simulink model "CubeX_LQR_2D"  (R2016b)
settings: Solver=FixedStepDiscrete  StartTime=0.0  StopTime=inf  FixedStep=0.002  RelTol=1e-3
PreLoadFcn:
  | waijung.modelPreload; % Required for working with Waijung Blockset. Do not remove.
InitFcn:
  | cubeparameters
values from neighbouring files (symbols this model uses):
  A = [0 0 0 0 0 0 0 0 0 0 283.190307038 0 ... (36 elements, 6x6)]    [K_lqr_3D.mat]
  C = [1 0 0 0 0 0 0 1 0 0 0 0 ... (36 elements, 6x6)]    [K_lqr_3D.mat]
  deg_ = 0.0174532925199    [K_lqr_3D.mat]
  g = 9.81    [K_lqr_3D.mat]
  imu =     [K_lqr_3D.mat]
  K_lqr = [204.402503892 25.7626324054]    [K_lqr_3D.mat]
  motor =     [K_lqr_3D.mat]
undefined symbols (not defined in the file or in its folder): Link, LQFP100, ST, STM32F407VG, STM32F4DISCOVERY
libraries: simulink x39, stm32f4_i2c_lib x8, stm32f4_io_lib x7, cube_lib x5, BC_USB x2, stm32f4_adc_lib x1, stm32f4_device_config_lib x1
(part 1 of 3)
CloseFcn:
  | waijung.modelClose; % Required for working with Waijung Blockset. Do not remove.
settings Model: Creator=Hi  LastModifiedBy=Wall
settings DataIOCC: LimitDataPoints=on  SaveFormat=Array
settings OptimizationCC: LifeSpan=1
settings DebuggingCC: AllowSymbolicDim=off  SFUnexpectedBacktrackingDiag=warning  SFNoUnconditionalDefaultTransitionDiag=warning  SFExecutionAtInitializationDiag=none
settings HardwareCC: ProdBitPerPointer=32  ProdBitPerSizeT=32  ProdBitPerPtrDiffT=32  ProdLargestAtomicFloat=None  ProdIntDivRoundTo=Undefined  ProdWordSize=32  ProdHWDeviceType=ARM Compatible->Cortex - M4  TargetEndianess=LittleEndian  TargetHWDeviceType=ARM Compatible->Cortex - M4
settings ModelReferenceCC: PropagateSignalLabelsOutOfModel=off
settings RTWCC: SystemTargetFile=stm32f4.tlc  GenerateMakefile=off  TemplateMakefile=ert_default_tmf  Description=STM32F4 Target
settings CodeAppCC: ForceParamTrailComments=on  IgnoreCustomStorageClasses=off  OperatorAnnotations=on  SimulinkDataObjDesc=on  InsertBlockDesc=on  MATLABSourceComments=on
settings STFCustomTargetCC: ModelReferenceCompliant=off  CombineOutputUpdateFcns=on  ERTCustomFileBanners=on  SupportContinuousTime=off  SupportNonInlinedSFcns=off  RemoveResetFunc=on  MATLABClassNameForMDSCustomization=Simulink.SoftwareTarget.ERTCustomization  GRTInterface=off  SystemTargetFile=stm32f4.tlc
settings ERTTargetCC: ModelReferenceCompliant=off  ParMdlRefBuildCompliant=off  CompOptLevelCompliant=off  ConcurrentExecutionCompliant=off  ERTFirstTimeCompliant=off  ModelStepFunctionPrototypeControlCompliant=off  CPPClassGenCompliant=off  UseToolchainInfoCompliant=off  ERTSrcFileBannerTemplate=stm32f4_code_template.cgt  ERTHdrFileBannerTemplate=stm32f4_code_template.cgt  ERTDataSrcFileTemplate=stm32f4_code_template.cgt  ERTDataHdrFileTemplate=stm32f4_code_template.cgt  ERTCustomFileTemplate=stm32f4_file_process.tlc  ConvertIfToSwitch=off  SuppressUnreachableDefaultCases=off
settings ConfigComp: CovMetricSettings=dw  CovHtmlReporting=on  CovSaveCumulativeToWorkspaceVar=on  CovSaveSingleToWorkspaceVar=on  CovExternalEMLEnable=off

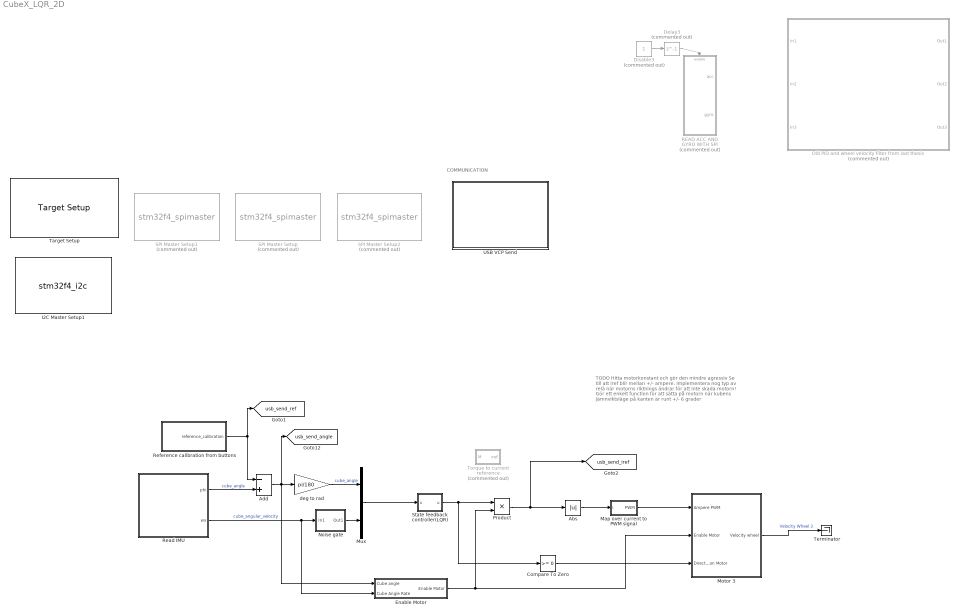
== system CubeX_LQR_2D ==
  note: TODO
      | Hitta motorkonstant och gör den mindre agressiv
      | Se till att iref blir mellan +/- ampere.
      |
      | Implementera nog typ av relä när motorns riktnings
      | ändrar för att inte skada motorn!
      |
      | Gör ett enkelt function för att sätta på motorn när kubens
      | jämnviktsläge på kanten är runt +/- 6 grader
  note: COMMUNICATION
  Abs : Abs
  Add : Sum  Inputs=-+
  Compare To Zero : simulink/Logic and Bit Operations/Compare To Zero  relop=>=  OutDataTypeStr=boolean
  Delay3 : Delay  Commented=on  DelayLength=1  InitialCondition=0
  Disable3 : Constant  Commented=on
  Enable Motor : Subsystem
  I2C Master Setup1 : S-Function  FunctionName=stm32f4_i2c  Parameters=configuration,module,transfer,clkspeed,timeout,sdapin,sclpin,writecount,readcount,inputtypearray,outputtypearray,confstr,sampletime,sampletimestr,blockid  SFunctionDeploymentMode=off  EnableBusSupport=off  mask(stm32f4_i2c){configuration=Setup, module=1, lastmodule=1, transfer=Blocking, dutycycle=TLow/THigh = 2, clkspeed=400, timeout=25, writecount=0, readcount=0, sdapin=B9, sclpin=B6, waitwritetime=0, inputtypearray=[0], outputtypearray=[0], confstr=["B","9","B","6","1","1","6","0","I2C_DutyCycle_2","0","off"], sampletime=-1, sampletimestr=0.002, blockid=I2CMasterSetup1}
      mask prompts: module "I2C Module"; lastmodule "Last module"; transfer "Transfer mode"; dutycycle "Duty cycle in fast mode"; clkspeed "Clock speed (kHz)"; timeout "Timeout (ms)"; writecount "Bytes write count"; readcount "Bytes read count"; sdapin "SDA pin"; sclpin "SCL pin"; waitwritetime "Wait write time (ms), default is 0"; inputtypearray "Input type array"; outputtypearray "Output type array"; confstr "Configuration string"; sampletime "Sample time (sec)"; sampletimestr "Compiled sample time (sec) in string"
      mask init:
      | stm32f4_i2c_callback('init');
      mask Help: web(fullfile(waijungdocroot,'stm32f4_i2c_setup.htm'), '-browser')
      mask TypeOptions configuration: Setup | Transaction
      mask Callback configuration: stm32f4_i2c_callback('configuration');
      mask TypeOptions module: 1 | 2 | 3
      mask Callback module: stm32f4_i2c_callback('module');
      mask TypeOptions transfer: Blocking | Non-blocking
      mask TypeOptions dutycycle: TLow/THigh = 16/9 | TLow/THigh = 2
      mask Callback dutycycle: stm32f4_i2c_callback('dutycycle');
      mask Callback writecount: stm32f4_i2c_callback('writecount');
      mask Callback readcount: stm32f4_i2c_callback('readcount');
      mask TypeOptions sdapin: - | B7 | B9
      mask Callback sdapin: stm32f4_i2c_callback('sdapin');
      mask TypeOptions sclpin: - | B6 | B8
      mask Callback sclpin: stm32f4_i2c_callback('sclpin');
      mask Callback confstr: stm32f4_i2c_callback('confstr');
      mask Callback sampletime: stm32f4_i2c_callback('sampletime');
      mask Callback sampletimestr: stm32f4_i2c_callback('sampletimestr');
      mask Callback blockid: stm32f4_i2c_callback('blockid');
      mask Display: text(0.5, 0.5, 'Module: I2C1\nClock: 400kHz\nSDA/SCL Pin: B9/B6','ver','middle','hor','center');
  Map over current to PWM signal : Subsystem
  Motor 3 : Subsystem
  Mux : Mux  Inputs=2
  Noise gate : Subsystem
  Old PID and wheel velocity filter from last thesis : Subsystem  Commented=on
  Product : Product
  READ ACC AND GYRO WITH SPI : Subsystem  Commented=on
  Read IMU : Subsystem
  Reference calibration from buttons : Subsystem
  SPI Master Setup : S-Function  Commented=on  FunctionName=stm32f4_spimaster  Parameters=mode,configuration,module,datacount,inputtypearray,outputtypearray,confstr,sampletime,sampletimestr,blockid  SFunctionDeploymentMode=off  EnableBusSupport=off  mask(stm32f4_spimaster){configuration=Setup, module=2, mode=Write, lastmodule=2, direction=Full-Duplex, dataformat=8bit/ FirstBit_MSB, prescaler=32, lastpclk=42000000, baudrate=1312500, cpolcpha=CPOL_Low/ CPHA_1Edge, datacount=0, nssmode=Software, nsspin=Not used, softnssport=B, softnsspin=12, sckpin=B13, misopin=B14, mosipin=B15, pintype=Push Pull, pulltype=Pull Up, nssdelay=0, inputtypearray=[0], outputtypearray=[0], confstr=["SPI_Direction_2Lines_FullDuplex","8b","MSB","Low","1Edge","32","Soft","0","x","x","1","B","12","1","B","13","1","B","14","1","B","15","0","1","0","0","0","0","0","0","0","PP","0","UP"], sampletime=-1, sampletimestr=-1, blockid=SPIMasterSetup}
      mask prompts: module "SPI Module:"; lastmodule "Last module:"; dataformat "Data format:"; prescaler "Buad rate prescaler: Pclk/"; lastpclk "Last PCLK"; baudrate "Baud rate (Hz)"; cpolcpha "Clock polarity (CPOL)/ Clock phase (CPHA):"; datacount "Data Write count:"; nssmode "Slave/chip select (nSS, nCS) mode"; nsspin "Slave/chip select (nSS, nCS) pin"; softnssport "Slave/chip select port (nSS, nCS)"; softnsspin "Slave/chip select pin (nSS, nCS)"; sckpin "SCLK pin:"; misopin "MISO pin:"; mosipin "MOSI pin:"; pintype "Pin type (Push-Pull/Open-Drain)"; pulltype "Pull Type (Up/Down)"; nssdelay "Data delay time, uS:"; inputtypearray "Input type array"; outputtypearray "Output type array"; confstr "Configuration string"; sampletime "Sample time (sec)"; sampletimestr "Compiled sample time (sec) in string"
      mask help:
      | Direction:
      |  - Full-Duplex, use this mode when need to send and receive data at same clock.
      |  - Half-Duplex_Tx, this mode is to transmit data to slave only. Pin MISO (Rx) can be free for other function.
      |  - Half-Duplex_Rx, this mode is to receive data from slave only. Pin MOSIO (Tx) can be free for other function.
      | Data format:
      |   This configuration is depending on the specification of slave device.
      | Baud rate prescaler:
      |  - Use this prescaler to devide from the PCLK for SPI clock.
      |  - This Prescaler value is auto determine corresponding to baudrate setting and selected SPI module.
      | Baud rate (Hz):
      |  - Select baud rate for SPI clock. Please check the maximum clock support for target slave device.
      | Clock polarity and Clock phase:
      |  - This configuration parameter is depending on slave device.
      |  - See waijung help for more description.
      | Slave/chip select mode:
      |  - Hardware, use hardware SPI module for slave select (or chip select) pin.
      |  - Software, this mode allow any available pin for slave select (or chip select) function.
      |  - Custom, SPI block did not control slave select pin. User may use Digital Output block to control by costom.
      mask init:
      | stm32f4_spimaster_callback('init');
      mask Help: web(fullfile(waijungdocroot,'stm32f4_spimaster_setup.htm'), '-browser')
      mask TypeOptions configuration: Setup | Transaction
      mask Callback configuration: stm32f4_spimaster_callback('configuration');
      mask TypeOptions module: 1 | 2 | 3
      mask Callback module: stm32f4_spimaster_callback('module');
      mask TypeOptions mode: Read/ Write | Read | Write
      mask Callback mode: stm32f4_spimaster_callback('mode');
      mask TypeOptions direction: Full-Duplex | Half-Duplex_Tx | Half-Duplex_Rx
      mask Callback direction: stm32f4_spimaster_callback('direction');
      mask TypeOptions dataformat: 8bit/ FirstBit_MSB | 8bit/ FirstBit_LSB | 16bit/ FirstBit_MSB | 16bit/ FirstBit_LSB
      mask TypeOptions prescaler: 2 | 4 | 8 | 16 | 32 | 64 | 128 | 256
      mask TypeOptions baudrate: Not set | 21000000 | 10500000 | 5250000 | 2625000 | 1312500 | 656250 | 328125 | 164063
      mask Callback baudrate: stm32f4_spimaster_callback('baudrate');
      mask TypeOptions cpolcpha: CPOL_Low/ CPHA_1Edge | CPOL_Low/ CPHA_2Edge | CPOL_High/ CPHA_1Edge | CPOL_High/ CPHA_2Edge
      mask Callback datacount: stm32f4_spimaster_callback('datacount');
      mask TypeOptions nssmode: Hardware | Software | Custom
      mask Callback nssmode: stm32f4_spimaster_callback('nssmode');
      mask TypeOptions nsspin: Not used | B9 | B12
      mask TypeOptions softnssport: A | B | C | D | E | F | G | H | I
      mask TypeOptions softnsspin: 0 | 1 | 2 | 3 | 4 | 5 | 6 | 7 | 8 | 9 | 10 | 11 | 12 | 13 | 14 | 15
      mask TypeOptions sckpin: Not used | B10 | B13
      mask TypeOptions misopin: Not used | B14 | C2
      mask TypeOptions mosipin: Not used | B15 | C3
      mask TypeOptions pintype: Push Pull | Open Drain
      mask TypeOptions pulltype: None | Pull Up | Pull Down
      mask Callback confstr: stm32f4_spimaster_callback('confstr');
      mask Callback sampletime: stm32f4_spimaster_callback('sampletime');
      mask Callback sampletimestr: stm32f4_spimaster_callback('sampletimestr');
      mask Callback blockid: stm32f4_spimaster_callback('blockid');
      mask Display: text(0.5, 0.5, 'Module: SPI2 (Master)\nFull-Duplex\nBaudrate: 1312500','ver','middle','hor','center');
  SPI Master Setup1 : S-Function  Commented=on  FunctionName=stm32f4_spimaster  Parameters=mode,configuration,module,datacount,inputtypearray,outputtypearray,confstr,sampletime,sampletimestr,blockid  SFunctionDeploymentMode=off  EnableBusSupport=off  mask(stm32f4_spimaster){configuration=Setup, module=1, mode=Write, lastmodule=1, direction=Full-Duplex, dataformat=8bit/ FirstBit_MSB, prescaler=64, lastpclk=84000000, baudrate=1312500, cpolcpha=CPOL_Low/ CPHA_1Edge, datacount=0, nssmode=Software, nsspin=Not used, softnssport=C, softnsspin=5, sckpin=A5, misopin=A6, mosipin=A7, pintype=Push Pull, pulltype=Pull Up, nssdelay=0, inputtypearray=[0], outputtypearray=[0], confstr=["SPI_Direction_2Lines_FullDuplex","8b","MSB","Low","1Edge","64","Soft","0","x","x","1","C","5","1","A","5","1","A","6","1","A","7","1","0","1","0","0","0","0","0","0","PP","0","UP"], sampletime=-1, sampletimestr=-1, blockid=SPIMasterSetup1}
      mask prompts: module "SPI Module:"; lastmodule "Last module:"; dataformat "Data format:"; prescaler "Buad rate prescaler: Pclk/"; lastpclk "Last PCLK"; baudrate "Baud rate (Hz)"; cpolcpha "Clock polarity (CPOL)/ Clock phase (CPHA):"; datacount "Data Write count:"; nssmode "Slave/chip select (nSS, nCS) mode"; nsspin "Slave/chip select (nSS, nCS) pin"; softnssport "Slave/chip select port (nSS, nCS)"; softnsspin "Slave/chip select pin (nSS, nCS)"; sckpin "SCLK pin:"; misopin "MISO pin:"; mosipin "MOSI pin:"; pintype "Pin type (Push-Pull/Open-Drain)"; pulltype "Pull Type (Up/Down)"; nssdelay "Data delay time, uS:"; inputtypearray "Input type array"; outputtypearray "Output type array"; confstr "Configuration string"; sampletime "Sample time (sec)"; sampletimestr "Compiled sample time (sec) in string"
      mask help:
      | Direction:
      |  - Full-Duplex, use this mode when need to send and receive data at same clock.
      |  - Half-Duplex_Tx, this mode is to transmit data to slave only. Pin MISO (Rx) can be free for other function.
      |  - Half-Duplex_Rx, this mode is to receive data from slave only. Pin MOSIO (Tx) can be free for other function.
      | Data format:
      |   This configuration is depending on the specification of slave device.
      | Baud rate prescaler:
      |  - Use this prescaler to devide from the PCLK for SPI clock.
      |  - This Prescaler value is auto determine corresponding to baudrate setting and selected SPI module.
      | Baud rate (Hz):
      |  - Select baud rate for SPI clock. Please check the maximum clock support for target slave device.
      | Clock polarity and Clock phase:
      |  - This configuration parameter is depending on slave device.
      |  - See waijung help for more description.
      | Slave/chip select mode:
      |  - Hardware, use hardware SPI module for slave select (or chip select) pin.
      |  - Software, this mode allow any available pin for slave select (or chip select) function.
      |  - Custom, SPI block did not control slave select pin. User may use Digital Output block to control by costom.
      mask init:
      | stm32f4_spimaster_callback('init');
      mask Help: web(fullfile(waijungdocroot,'stm32f4_spimaster_setup.htm'), '-browser')
      mask TypeOptions configuration: Setup | Transaction
      mask Callback configuration: stm32f4_spimaster_callback('configuration');
      mask TypeOptions module: 1 | 2 | 3
      mask Callback module: stm32f4_spimaster_callback('module');
      mask TypeOptions mode: Read/ Write | Read | Write
      mask Callback mode: stm32f4_spimaster_callback('mode');
      mask TypeOptions direction: Full-Duplex | Half-Duplex_Tx | Half-Duplex_Rx
      mask Callback direction: stm32f4_spimaster_callback('direction');
      mask TypeOptions dataformat: 8bit/ FirstBit_MSB | 8bit/ FirstBit_LSB | 16bit/ FirstBit_MSB | 16bit/ FirstBit_LSB
      mask TypeOptions prescaler: 2 | 4 | 8 | 16 | 32 | 64 | 128 | 256
      mask TypeOptions baudrate: Not set | 42000000 | 21000000 | 10500000 | 5250000 | 2625000 | 1312500 | 656250 | 328125
      mask Callback baudrate: stm32f4_spimaster_callback('baudrate');
      mask TypeOptions cpolcpha: CPOL_Low/ CPHA_1Edge | CPOL_Low/ CPHA_2Edge | CPOL_High/ CPHA_1Edge | CPOL_High/ CPHA_2Edge
      mask Callback datacount: stm32f4_spimaster_callback('datacount');
      mask TypeOptions nssmode: Hardware | Software | Custom
      mask Callback nssmode: stm32f4_spimaster_callback('nssmode');
      mask TypeOptions nsspin: Not used | A4 | A15
      mask TypeOptions softnssport: A | B | C | D | E | F | G | H | I
      mask TypeOptions softnsspin: 0 | 1 | 2 | 3 | 4 | 5 | 6 | 7 | 8 | 9 | 10 | 11 | 12 | 13 | 14 | 15
      mask TypeOptions sckpin: Not used | A5 | B3
      mask TypeOptions misopin: Not used | A6 | B4
      mask TypeOptions mosipin: Not used | A7 | B5
      mask TypeOptions pintype: Push Pull | Open Drain
      mask TypeOptions pulltype: None | Pull Up | Pull Down
      mask Callback confstr: stm32f4_spimaster_callback('confstr');
      mask Callback sampletime: stm32f4_spimaster_callback('sampletime');
      mask Callback sampletimestr: stm32f4_spimaster_callback('sampletimestr');
      mask Callback blockid: stm32f4_spimaster_callback('blockid');
      mask Display: text(0.5, 0.5, 'Module: SPI1 (Master)\nFull-Duplex\nBaudrate: 1312500','ver','middle','hor','center');
  SPI Master Setup2 : S-Function  Commented=on  FunctionName=stm32f4_spimaster  Parameters=mode,configuration,module,datacount,inputtypearray,outputtypearray,confstr,sampletime,sampletimestr,blockid  SFunctionDeploymentMode=off  EnableBusSupport=off  mask(stm32f4_spimaster){configuration=Setup, module=3, mode=Write, lastmodule=3, direction=Full-Duplex, dataformat=8bit/ FirstBit_MSB, prescaler=32, lastpclk=42000000, baudrate=1312500, cpolcpha=CPOL_Low/ CPHA_1Edge, datacount=0, nssmode=Software, nsspin=Not used, softnssport=C, softnsspin=11, sckpin=C10, misopin=B4, mosipin=B5, pintype=Push Pull, pulltype=Pull Up, nssdelay=0, inputtypearray=[0], outputtypearray=[0], confstr=["SPI_Direction_2Lines_FullDuplex","8b","MSB","Low","1Edge","32","Soft","0","x","x","1","C","11","1","C","10","1","B","4","1","B","5","0","1","1","0","0","0","0","0","0","PP","0","UP"], sampletime=-1, sampletimestr=-1, blockid=SPIMasterSetup2}
      mask prompts: module "SPI Module:"; lastmodule "Last module:"; dataformat "Data format:"; prescaler "Buad rate prescaler: Pclk/"; lastpclk "Last PCLK"; baudrate "Baud rate (Hz)"; cpolcpha "Clock polarity (CPOL)/ Clock phase (CPHA):"; datacount "Data Write count:"; nssmode "Slave/chip select (nSS, nCS) mode"; nsspin "Slave/chip select (nSS, nCS) pin"; softnssport "Slave/chip select port (nSS, nCS)"; softnsspin "Slave/chip select pin (nSS, nCS)"; sckpin "SCLK pin:"; misopin "MISO pin:"; mosipin "MOSI pin:"; pintype "Pin type (Push-Pull/Open-Drain)"; pulltype "Pull Type (Up/Down)"; nssdelay "Data delay time, uS:"; inputtypearray "Input type array"; outputtypearray "Output type array"; confstr "Configuration string"; sampletime "Sample time (sec)"; sampletimestr "Compiled sample time (sec) in string"
      mask help:
      | Direction:
      |  - Full-Duplex, use this mode when need to send and receive data at same clock.
      |  - Half-Duplex_Tx, this mode is to transmit data to slave only. Pin MISO (Rx) can be free for other function.
      |  - Half-Duplex_Rx, this mode is to receive data from slave only. Pin MOSIO (Tx) can be free for other function.
      | Data format:
      |   This configuration is depending on the specification of slave device.
      | Baud rate prescaler:
      |  - Use this prescaler to devide from the PCLK for SPI clock.
      |  - This Prescaler value is auto determine corresponding to baudrate setting and selected SPI module.
      | Baud rate (Hz):
      |  - Select baud rate for SPI clock. Please check the maximum clock support for target slave device.
      | Clock polarity and Clock phase:
      |  - This configuration parameter is depending on slave device.
      |  - See waijung help for more description.
      | Slave/chip select mode:
      |  - Hardware, use hardware SPI module for slave select (or chip select) pin.
      |  - Software, this mode allow any available pin for slave select (or chip select) function.
      |  - Custom, SPI block did not control slave select pin. User may use Digital Output block to control by costom.
      mask init:
      | stm32f4_spimaster_callback('init');
      mask Help: web(fullfile(waijungdocroot,'stm32f4_spimaster_setup.htm'), '-browser')
      mask TypeOptions configuration: Setup | Transaction
      mask Callback configuration: stm32f4_spimaster_callback('configuration');
      mask TypeOptions module: 1 | 2 | 3
      mask Callback module: stm32f4_spimaster_callback('module');
      mask TypeOptions mode: Read/ Write | Read | Write
      mask Callback mode: stm32f4_spimaster_callback('mode');
      mask TypeOptions direction: Full-Duplex | Half-Duplex_Tx | Half-Duplex_Rx
      mask Callback direction: stm32f4_spimaster_callback('direction');
      mask TypeOptions dataformat: 8bit/ FirstBit_MSB | 8bit/ FirstBit_LSB | 16bit/ FirstBit_MSB | 16bit/ FirstBit_LSB
      mask TypeOptions prescaler: 2 | 4 | 8 | 16 | 32 | 64 | 128 | 256
      mask TypeOptions baudrate: Not set | 21000000 | 10500000 | 5250000 | 2625000 | 1312500 | 656250 | 328125 | 164063
      mask Callback baudrate: stm32f4_spimaster_callback('baudrate');
      mask TypeOptions cpolcpha: CPOL_Low/ CPHA_1Edge | CPOL_Low/ CPHA_2Edge | CPOL_High/ CPHA_1Edge | CPOL_High/ CPHA_2Edge
      mask Callback datacount: stm32f4_spimaster_callback('datacount');
      mask TypeOptions nssmode: Hardware | Software | Custom
      mask Callback nssmode: stm32f4_spimaster_callback('nssmode');
      mask TypeOptions nsspin: Not used | A4 | A15
      mask TypeOptions softnssport: A | B | C | D | E | F | G | H | I
      mask TypeOptions softnsspin: 0 | 1 | 2 | 3 | 4 | 5 | 6 | 7 | 8 | 9 | 10 | 11 | 12 | 13 | 14 | 15
      mask TypeOptions sckpin: Not used | B3 | C10
      mask TypeOptions misopin: Not used | B4 | C11
      mask TypeOptions mosipin: Not used | B5 | C12
      mask TypeOptions pintype: Push Pull | Open Drain
      mask TypeOptions pulltype: None | Pull Up | Pull Down
      mask Callback confstr: stm32f4_spimaster_callback('confstr');
      mask Callback sampletime: stm32f4_spimaster_callback('sampletime');
      mask Callback sampletimestr: stm32f4_spimaster_callback('sampletimestr');
      mask Callback blockid: stm32f4_spimaster_callback('blockid');
      mask Display: text(0.5, 0.5, 'Module: SPI3 (Master)\nFull-Duplex\nBaudrate: 1312500','ver','middle','hor','center');
  State feedback controller(LQR) : Subsystem
      settings: MinAlgLoopOccurrences=on
  Target Setup : stm32f4_device_config_lib/Target Setup  Priority=100  compiler=GNU ARM  previous_compiler=GNU ARM  mcu=STM32F407VG (LQFP100); STM32F4DISCOVERY  mcustr=STM32F407VG  clockconfig=STM32F4DISCOVERY Default (HSEOSC-8MHz/HCLK-168MHz)  system_stm32f4xx_c_path=C:\waijung15_04a\targets\stm32f4_target\stm32f4\utils\STM32F4xx_AN3988_V1.0.1\stm32f4_default\hseosc8mhz  showmemoryconfiguration=off  stacksize=0x400  heapsize=0x200  enableautocompiledownload=on  fullchiperase=off  programmerinterface=ST-Link  editctrlstr=on  compilercontrolstr=$(patsubst %, -I%, .) -mcpu=cortex-m4 -mthumb -mthumb-interwork -mfloat-abi=hard -mfpu=fpv4-sp-d16 -ffast-math -Wall -Wextra -Ofast  assemblercontrolstr=$(patsubst %, -I%, .) -mcpu=cortex-m4 -mthumb -mthumb-interwork -mfloat-abi=hard -mfpu=fpv4-sp-d16 -ffast-math -Wall -Wextra -Ofast -Wa,-amhls=$(<:.s=.lst) -D__STACK_SIZE=$(STACK_SIZE) -D__HEAP_SIZE=$(HEAP_SIZE)  linkercontrolstr=-T$(LD_SCRIPT) -g -Wl,-Map=$(MAP),--cref,--no-warn-mismatch -mcpu=cortex-m4 -mthumb -mthumb-interwork -mfloat-abi=hard -mfpu=fpv4-sp-d16  runafterdownload=on  execprofile=None  profileruart=1  profilerbaud=115200  profilertxpin=Not used  profilerinitstr=0.002,168000000,336000,115200,0  manualsetsampletime=on  sampletime=0.002  blockid=TargetSetup  systickreloadvalue=336000  hseval=8000000  lastprofileruart=1  hclk=168000000  flashorigin=0x8000000  flashlength=1M  ramorigin=0x20000000  ramlength=112k  useextram=off
  Terminator : Terminator
  Torque to current reference : Subsystem  Commented=on
  USB VCP Send : Subsystem
  deg to rad : Gain  Gain=pi/180
  tag scope: usb_send_angle=global, usb_send_iref=global, usb_send_ref=global
  wires:
  Disable3/1 -> Delay3/1
  Delay3/1 -> READ ACC AND GYRO WITH SPI/Enable
  Read IMU/2(wx) -> Noise gate/1(In1), Enable Motor/2(Cube Angle Rate)  "cube_angular_velocity"
  Reference calibration from buttons/1(reference_calibration) -> [usb_send_ref], Add/1
  Read IMU/1(phi) -> Add/2  "cube_angle"
  Map over current to PWM signal/1(PWM) -> Motor 3/1(Ampere PWM)
  Add/1 -> Enable Motor/1(Cube angle), [usb_send_angle], deg to rad/1
  deg to rad/1 -> Mux/1  "cube_angle"
  State feedback controller(LQR)/1(u) -> Product/1, Compare To Zero/1
  Motor 3/1(Velocity wheel) -> Terminator/1  "Velocity Wheel 3"
  Abs/1 -> Map over current to PWM signal/1(i)
  Mux/1 -> State feedback controller(LQR)/1(x)
  Enable Motor/1(Enable Motor) -> Product/2, Motor 3/2(Enable Motor)
  Compare To Zero/1 -> Motor 3/3("Direction Motor ")
  Product/1 -> [usb_send_iref], Abs/1
  Noise gate/1(Out1) -> Mux/2

== system CubeX_LQR_2D/Enable Motor ==
  note: When the angle is abs of 6 degrees, Motor is enabled
  Cube angle : Inport
  Cube Angle Rate : Inport  Port=2
  Abs : Abs
  Abs1 : Abs
  Compare To Constant : simulink/Logic and Bit Operations/Compare To Constant  relop=<=  const=4  OutDataTypeStr=boolean
  Compare To Constant1 : simulink/Logic and Bit Operations/Compare To Constant  Commented=through  relop=>=  const=0.05  OutDataTypeStr=boolean
  Compare To Constant2 : simulink/Logic and Bit Operations/Compare To Constant  relop=>=  const=0.035  OutDataTypeStr=boolean
  Constant : Constant
  Logical Operator : Logic  AllPortsSameDT=off  OutDataTypeStr=boolean
  Terminator : Terminator
  Enable Motor : Outport
  wires:
  Abs1/1 -> Compare To Constant1/1, Compare To Constant/1
  Cube angle/1 -> Abs1/1
  Compare To Constant/1 -> Logical Operator/1
  Logical Operator/1 -> Enable Motor/1
  Cube Angle Rate/1 -> Abs/1
  Abs/1 -> Compare To Constant2/1
  Compare To Constant2/1 -> Terminator/1
  Constant/1 -> Logical Operator/2

== system CubeX_LQR_2D/Map over current to PWM signal ==
  note: Map over current to duty
      | current limit: 0-4A
      | duty limit: 10-90%
      |
      | (90-10) / (4-0) = 20 -> k
      | 10 -> m
  i : Inport
  Add : Sum
  Saturation on duty : Saturate  UpperLimit=90  LowerLimit=10
  k : Constant  Value=10
  m : Gain  Gain=20
  PWM : Outport
  wires:
  k/1 -> Add/1
  Add/1 -> Saturation on duty/1
  m/1 -> Add/2
  i/1 -> m/1
  Saturation on duty/1 -> PWM/1

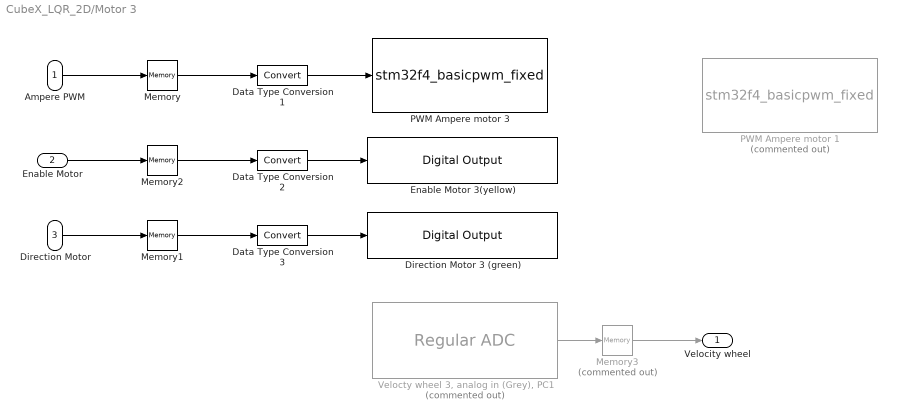
== system CubeX_LQR_2D/Motor 3 ==
  Ampere PWM : Inport
  Enable Motor : Inport  Port=2
  "Direction Motor " : Inport  Port=3
  Data Type Conversion1 : DataTypeConversion
  Data Type Conversion2 : DataTypeConversion
  Data Type Conversion3 : DataTypeConversion
  Direction Motor 3 (green) : stm32f4_io_lib/Digital Output  use_bitband=on  port=D  speed=100  porttype=Push Pull  porttypestr=PP  use_pin0=off  use_pin1=off  use_pin2=off  use_pin3=off  use_pin4=off  use_pin5=off  use_pin6=off  use_pin7=off  use_pin8=off  use_pin9=off  use_pin10=off  use_pin11=on  use_pin12=off  use_pin13=off  use_pin14=off  use_pin15=off  pinstr=GPIO_Pin_11  usedpinarray="[0  0  0  0  0  0  0  0  0  0  0  1  0  0  0  0]"  bitbandingstr="#define Motor3DirectionMotor3green_D11 Peripheral_BB(GPIOD->ODR, 11)  /* Output pin */"  sampletime=-1  sampletimestr=0.002  blockid=Motor3DirectionMotor3green  enablecustomportlabel=off  globalinit=off  cinputportlabel=In1, In2  coutputportlabel=0
  Enable Motor 3(yellow) : stm32f4_io_lib/Digital Output  use_bitband=on  port=D  speed=100  porttype=Push Pull  porttypestr=PP  use_pin0=off  use_pin1=off  use_pin2=off  use_pin3=off  use_pin4=off  use_pin5=off  use_pin6=off  use_pin7=off  use_pin8=off  use_pin9=on  use_pin10=off  use_pin11=off  use_pin12=off  use_pin13=off  use_pin14=off  use_pin15=off  pinstr=GPIO_Pin_9  usedpinarray="[0  0  0  0  0  0  0  0  0  1  0  0  0  0  0  0]"  bitbandingstr="#define Motor3EnableMotor3yellow_D9 Peripheral_BB(GPIOD->ODR, 9)  /* Output pin */"  sampletime=-1  sampletimestr=0.002  blockid=Motor3EnableMotor3yellow  enablecustomportlabel=off  globalinit=off  cinputportlabel=In1, In2  coutputportlabel=0
  Memory : Memory  InheritSampleTime=on
  Memory1 : Memory  InheritSampleTime=on
  Memory2 : Memory  InheritSampleTime=on
  Memory3 : Memory  Commented=on  InheritSampleTime=on
  PWM Ampere motor 1 : S-Function  Commented=on  FunctionName=stm32f4_basicpwm_fixed  Parameters=timer,pwmperiod,uc3m_pwmperiod,ch1pin,ch2pin,ch3pin,ch4pin,sampletime,sampletimestr,blockid,apb,portstr,pinstr,pinmat,timarr,timprescale,chmat,polaritystr  SFunctionDeploymentMode=off  EnableBusSupport=off  mask(stm32f4_basicpwm_fixed){timer=5, pwmperiod=0.02, uc3m_pwmperiod=0.0002, polarity=Active High, polaritystr=TIM_OCPolarity_High, ch1pin=Not available - Do not use, ch2pin=Not available - Do not use, ch3pin=Not available - Do not use, ch4pin=A3, sampletime=0.002, sampletimestr=0.002, blockid=motor3PWMAmperemotor3, portpinstr=,,,A3, enablecustomportlabel=off, cinputportlabel=In1, In2, In3, In4, coutputportlabel=0, callbackgensrccode=off, apb=1, portstr=["A"], pinstr=["GPIO_Pin_3"], pinmat=[1 3], timarr=59999, timprescale=55, chmat=[4]}
      mask prompts: pwmperiod "PWM Period (seconds)"; uc3m_pwmperiod "PWM Signal Period (seconds)"; ch1pin "Channel 1"; ch2pin "Channel 2"; ch3pin "Channel 3"; ch4pin "Channel 4"; sampletime "Sample time (sec)"; sampletimestr "Compiled sample time (sec) in string"; portpinstr "Port pin string"; enablecustomportlabel "Enable custom port labels"; cinputportlabel "Custom input port labels (Ex. In1, In2, In3)"; coutputportlabel "Custom output port labels (Ex. Out1, Out2, Out3)"; callbackgensrccode "Gen source code from callback"; portstr "Port string"; pinstr "Pin string"; pinmat "Pin matrix"; timarr "Timer ARR"; timprescale "Timer PRESCALE"; chmat "Channel order"
      mask help:
      | This block implements basic Edge-aligned Pulse Width Modulation (PWM) generation.
      | All timers are 16-bit. The PWM period is fixed (per timer).
      |
      | This block was fixed by Sr Antonio
      mask init:
      | stm32f4_basicpwm_callback_fixed('init');
      mask Help: web(fullfile(waijungdocroot,'stm32f4_basicpwm.htm'),'-browser')
      mask TypeOptions timer: 1 | 2 | 3 | 4 | 5 | 8 | 9 | 10 | 11 | 12 | 13 | 14
      mask Callback timer: stm32f4_basicpwm_callback_fixed('timer');
      mask Callback pwmperiod: stm32f4_basicpwm_callback_fixed('pwmperiod');
      mask Callback uc3m_pwmperiod: stm32f4_basicpwm_callback_fixed('uc3m_pwmperiod');
      mask TypeOptions polarity: Active High | Active Low
      mask Callback polarity: stm32f4_basicpwm_callback_fixed('polarity');
      mask TypeOptions ch1pin: Not available - Do not use | A0 | A5
      mask Callback ch1pin: stm32f4_basicpwm_callback_fixed('ch1pin');
      mask TypeOptions ch2pin: Not available - Do not use | A1 | B3
      mask Callback ch2pin: stm32f4_basicpwm_callback_fixed('ch2pin');
      mask TypeOptions ch3pin: Not available - Do not use | A2 | B10
      mask Callback ch3pin: stm32f4_basicpwm_callback_fixed('ch3pin');
      mask TypeOptions ch4pin: Not available - Do not use | A3 | B11
      mask Callback ch4pin: stm32f4_basicpwm_callback_fixed('ch4pin');
      mask Callback sampletime: stm32f4_basicpwm_callback_fixed('sampletime');
      mask Callback sampletimestr: stm32f4_basicpwm_callback_fixed('sampletimestr');
      mask Callback blockid: stm32f4_basicpwm_callback_fixed('blockid');
      mask Callback enablecustomportlabel: stm32f4_basicpwm_callback_fixed('enablecustomportlabel')
      mask Display: text(0.95, 0.5, 'UC3M FIXED\nTimer: 5\nPolarity: Active High\nPeriod (sec): 0.0002\nTs (sec): 0.002','ver','middle','hor','right');port_label('input', 1,'CH4 (A3)')
  PWM Ampere motor 3 : S-Function  FunctionName=stm32f4_basicpwm_fixed  Parameters=timer,pwmperiod,uc3m_pwmperiod,ch1pin,ch2pin,ch3pin,ch4pin,sampletime,sampletimestr,blockid,apb,portstr,pinstr,pinmat,timarr,timprescale,chmat,polaritystr  SFunctionDeploymentMode=off  EnableBusSupport=off  mask(stm32f4_basicpwm_fixed){timer=2, pwmperiod=0.02, uc3m_pwmperiod=0.0002, polarity=Active High, polaritystr=TIM_OCPolarity_High, ch1pin=Not available - Do not use, ch2pin=Not available - Do not use, ch3pin=Not available - Do not use, ch4pin=A3, sampletime=0.002, sampletimestr=0.002, blockid=Motor3PWMAmperemotor3, portpinstr=,,,A3, enablecustomportlabel=off, cinputportlabel=In1, In2, In3, In4, coutputportlabel=0, callbackgensrccode=off, apb=1, portstr=["A"], pinstr=["GPIO_Pin_3"], pinmat=[1 3], timarr=59999, timprescale=55, chmat=[4]}
      mask prompts: pwmperiod "PWM Period (seconds)"; uc3m_pwmperiod "PWM Signal Period (seconds)"; ch1pin "Channel 1"; ch2pin "Channel 2"; ch3pin "Channel 3"; ch4pin "Channel 4"; sampletime "Sample time (sec)"; sampletimestr "Compiled sample time (sec) in string"; portpinstr "Port pin string"; enablecustomportlabel "Enable custom port labels"; cinputportlabel "Custom input port labels (Ex. In1, In2, In3)"; coutputportlabel "Custom output port labels (Ex. Out1, Out2, Out3)"; callbackgensrccode "Gen source code from callback"; portstr "Port string"; pinstr "Pin string"; pinmat "Pin matrix"; timarr "Timer ARR"; timprescale "Timer PRESCALE"; chmat "Channel order"
      mask help:
      | This block implements basic Edge-aligned Pulse Width Modulation (PWM) generation.
      | All timers are 16-bit. The PWM period is fixed (per timer).
      |
      | This block was fixed by Sr Antonio
      mask init:
      | stm32f4_basicpwm_callback_fixed('init');
      mask Help: web(fullfile(waijungdocroot,'stm32f4_basicpwm.htm'),'-browser')
      mask TypeOptions timer: 1 | 2 | 3 | 4 | 5 | 8 | 9 | 10 | 11 | 12 | 13 | 14
      mask Callback timer: stm32f4_basicpwm_callback_fixed('timer');
      mask Callback pwmperiod: stm32f4_basicpwm_callback_fixed('pwmperiod');
      mask Callback uc3m_pwmperiod: stm32f4_basicpwm_callback_fixed('uc3m_pwmperiod');
      mask TypeOptions polarity: Active High | Active Low
      mask Callback polarity: stm32f4_basicpwm_callback_fixed('polarity');
      mask TypeOptions ch1pin: Not available - Do not use | A0 | A5
      mask Callback ch1pin: stm32f4_basicpwm_callback_fixed('ch1pin');
      mask TypeOptions ch2pin: Not available - Do not use | A1 | B3
      mask Callback ch2pin: stm32f4_basicpwm_callback_fixed('ch2pin');
      mask TypeOptions ch3pin: Not available - Do not use | A2 | B10
      mask Callback ch3pin: stm32f4_basicpwm_callback_fixed('ch3pin');
      mask TypeOptions ch4pin: Not available - Do not use | A3 | B11
      mask Callback ch4pin: stm32f4_basicpwm_callback_fixed('ch4pin');
      mask Callback sampletime: stm32f4_basicpwm_callback_fixed('sampletime');
      mask Callback sampletimestr: stm32f4_basicpwm_callback_fixed('sampletimestr');
      mask Callback blockid: stm32f4_basicpwm_callback_fixed('blockid');
      mask Callback enablecustomportlabel: stm32f4_basicpwm_callback_fixed('enablecustomportlabel')
      mask Display: text(0.95, 0.5, 'UC3M FIXED\nTimer: 2\nPolarity: Active High\nPeriod (sec): 0.0002\nTs (sec): 0.002','ver','middle','hor','right');port_label('input', 1,'CH4 (A3)')
  "Velocty wheel 3, analog in (Grey), PC1" : stm32f4_adc_lib/Regular ADC  Commented=on  adcmodule=3  outputdatatype=Double  prescaler=2  prescalerstr=ADC_Prescaler_Div2  chsamplingtime=Auto  chsamplingtimestr=ADC_SampleTime_480Cycles  read_an0=off  read_an1=off  read_an2=off  read_an3=off  read_an4=off  read_an5=off  read_an6=off  read_an7=off  read_an8=off  read_an9=off  read_an10=off  read_an11=on  read_an12=off  read_an13=off  read_an14=off  read_an15=off  read_an16=off  read_an17=off  read_an18=off  pinstr=GPIO_Pin_11  usedpinarray="[0  0  0  0  0  0  0  0  0  0  0  1  0  0  0  0  0  0  0]"  usedportidarray=[2]  usedpinidarray=[1]  usedpinidcount=1  sampletime=0.002  blockid=motor4Veloctywheel3analoginGreyPC1  enablecustomportlabel=off  cinputportlabel=0  coutputportlabel=Out1, Out2
  Velocity wheel : Outport
  wires:
  Ampere PWM/1 -> Memory/1
  Data Type Conversion3/1 -> Direction Motor 3 (green)/1
  Data Type Conversion2/1 -> Enable Motor 3(yellow)/1
  Memory/1 -> Data Type Conversion1/1
  Memory2/1 -> Data Type Conversion2/1
  "Direction Motor "/1 -> Memory1/1
  Memory1/1 -> Data Type Conversion3/1
  Enable Motor/1 -> Memory2/1
  "Velocty wheel 3, analog in (Grey), PC1"/1 -> Memory3/1
  Memory3/1 -> Velocity wheel/1
  Data Type Conversion1/1 -> PWM Ampere motor 3/1

== system CubeX_LQR_2D/Noise gate ==
  In1 : Inport
  Abs1 : Abs
  Compare To Constant : simulink/Logic and Bit Operations/Compare To Constant  relop=>=  const=0.05  OutDataTypeStr=boolean
  Product : Product
  Out1 : Outport
  wires:
  Abs1/1 -> Compare To Constant/1
  In1/1 -> Product/2, Abs1/1
  Product/1 -> Out1/1
  Compare To Constant/1 -> Product/1

== system CubeX_LQR_2D/Old PID and wheel velocity filter from last thesis ==
  In1 : Inport
  In2 : Inport  Port=2
  In3 : Inport  Port=3
  Filetered Wheel 3 : Subsystem  Commented=on
  "PID Motor 3 DONE " : Subsystem  Commented=on
  Out1 : Outport
  Out2 : Outport  Port=2
  Out3 : Outport  Port=3
  wires:
  In1/1 -> "PID Motor 3 DONE "/1("Welocity Wheel ")
  "PID Motor 3 DONE "/2("Direction_Motor_3 ") -> Out3/1
  In2/1 -> Filetered Wheel 3/1(In1)
  Filetered Wheel 3/1(Out1) -> Out2/1
  "PID Motor 3 DONE "/1(Motor_3_Out) -> Out1/1
  In3/1 -> "PID Motor 3 DONE "/2(Angle)
